simulink model "p1"  (R2020a)
settings: Solver=VariableStepAuto  StartTime=0.0  StopTime=0.08  RelTol=1e-3
model workspace (MAT data in the model file):
  b = Simulink.Parameter
  b.Value = 50
  b.DataType = 'auto'
  b.Dimensions = [1 1]
  k = Simulink.Parameter
  k.Value = 4
  k.DataType = 'auto'
  k.Dimensions = [1 1]
  k1 = Simulink.Parameter
  k1.Value = 50
  k1.DataType = 'auto'
  k1.Dimensions = [1 1]
  k12 = Simulink.Parameter
  k12.Value = 25
  k12.DataType = 'auto'
  k12.Dimensions = [1 1]
libraries: simulink x1
settings Model: OrderedModelArguments=off  Creator=007  LastModifiedBy=007

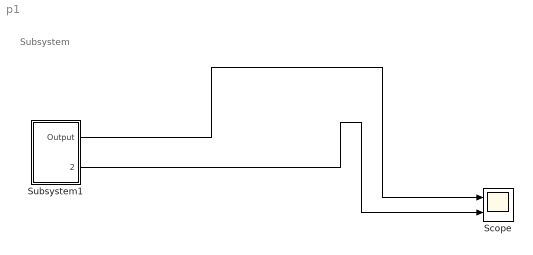
== system p1 ==
  note: Subsystem
  Scope : Scope  NumInputPorts=2
  Subsystem1 : Subsystem
  wires:
  Subsystem1/2(Output1) -> Scope/2
  Subsystem1/1(Output) -> Scope/1

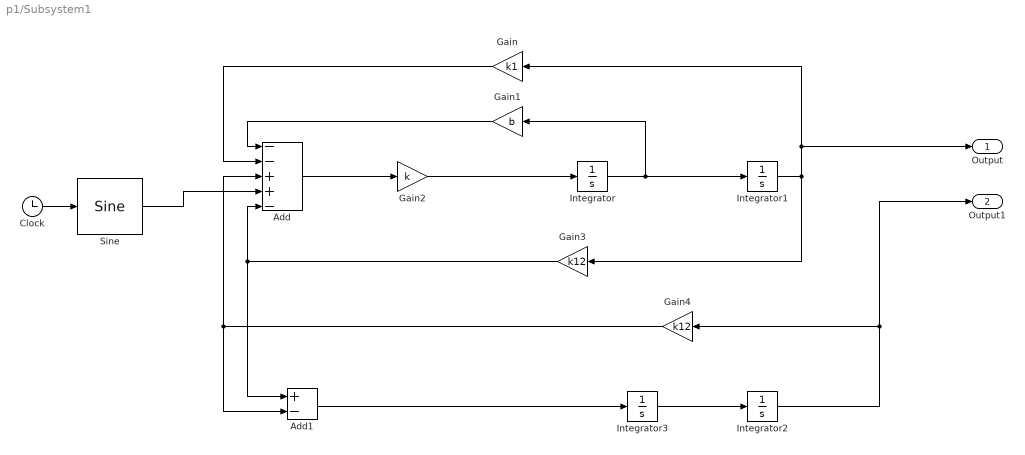
== system p1/Subsystem1 ==
  Add : Sum  Inputs=--++-
  Add1 : Sum  Inputs=+-
  Clock : Clock
  Gain : Gain  Gain=k1
  Gain1 : Gain  Gain=b
  Gain2 : Gain  Gain=k
  Gain3 : Gain  Gain=k12
  Gain4 : Gain  Gain=k12
  Integrator{,1..3} (4 alike) : Integrator
  Sine : simulink/Lookup Tables/Sine  Formula=sin(2*pi*u)  NumDataPoints=(2^5)+1  OutputWordLength=16  InternalRulePriority=Speed
  Output : Outport
  Output1 : Outport  Port=2
  wires:
  Gain3/1 -> Add1/1, Add/5
  Gain/1 -> Add/2
  Gain4/1 -> Add1/2, Add/3
  Integrator/1 -> Gain1/1, Integrator1/1
  Clock/1 -> Sine/1
  Add/1 -> Gain2/1
  Integrator3/1 -> Integrator2/1
  Integrator1/1 -> Gain3/1, Output/1, Gain/1
  Integrator2/1 -> Output1/1, Gain4/1
  Gain1/1 -> Add/1
  Add1/1 -> Integrator3/1
  Sine/1 -> Add/4
  Gain2/1 -> Integrator/1
